simulink model "ERLE"  (R2021b)
settings: Solver=VariableStepAuto  StartTime=0.0  StopTime=10.0  RelTol=1e-3
values from neighbouring files (symbols this model uses):
  T = 1    [Tempo.mat]
settings Model: Creator=jchav  LastModifiedBy=duart

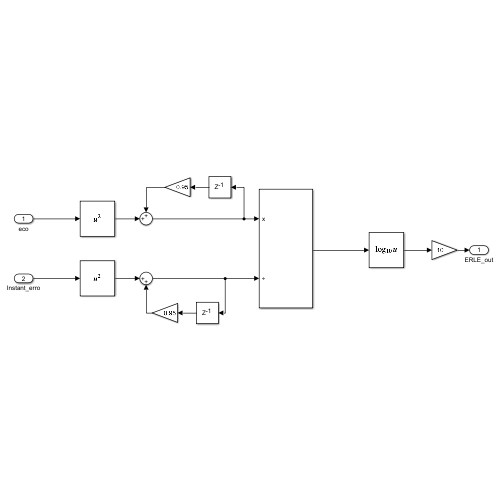
[thumbnail: Simulink's stored preview of the top-level diagram]
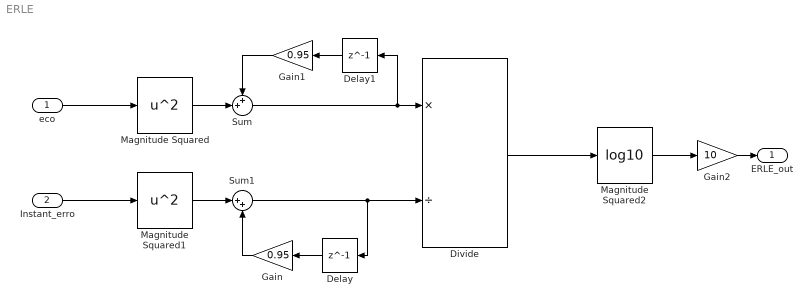
== system ERLE ==
  eco : Inport
  Instant_erro : Inport  Port=2
  Delay : Delay  DelayLength=1  InitialCondition=0  SampleTime=T
  Delay1 : Delay  DelayLength=1  InitialCondition=0  SampleTime=T
  Divide : Product  Inputs=*/
  Gain : Gain  Gain=0.95
  Gain1 : Gain  Gain=0.95
  Gain2 : Gain  Gain=10
  Magnitude Squared : Math  Operator=square  SaturateOnIntegerOverflow=on
  Magnitude Squared1 : Math  Operator=square  SaturateOnIntegerOverflow=on
  Magnitude Squared2 : Math  Operator=log10  SaturateOnIntegerOverflow=on
  Sum : Sum  Inputs=++|
  Sum1 : Sum  Inputs=|++
  ERLE_out : Outport
  wires:
  Instant_erro/1 -> Magnitude Squared1/1
  eco/1 -> Magnitude Squared/1
  Magnitude Squared1/1 -> Sum1/1
  Magnitude Squared/1 -> Sum/2
  Gain/1 -> Sum1/2
  Delay/1 -> Gain/1
  Sum1/1 -> Delay/1, Divide/2
  Gain1/1 -> Sum/1
  Sum/1 -> Delay1/1, Divide/1
  Delay1/1 -> Gain1/1
  Divide/1 -> Magnitude Squared2/1
  Magnitude Squared2/1 -> Gain2/1
  Gain2/1 -> ERLE_out/1
